simulink model "addSensorNoise"  (R2013a)
settings: Solver=ode45  StartTime=0.0  StopTime=10.0  RelTol=1e-3
values from neighbouring files (symbols this model uses):
  sampleTime = 0.01    [runPositionFilter.m]    (also in runtracklsq.m = mydata.sampleTime; workspace.mat)
libraries: simulink x9
settings Model: Creator=User  LastModifiedBy=User

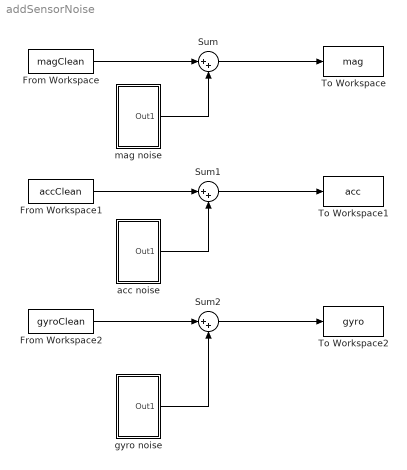
== system addSensorNoise ==
  From Workspace : FromWorkspace  VariableName=magClean  SampleTime=sampleTime
  From Workspace1 : FromWorkspace  VariableName=accClean  SampleTime=sampleTime
  From Workspace2 : FromWorkspace  VariableName=gyroClean  SampleTime=sampleTime
  Sum : Sum  Inputs=|++
  Sum1 : Sum  Inputs=|++
  Sum2 : Sum  Inputs=|++
  To Workspace : ToWorkspace  VariableName=mag  SampleTime=sampleTime  SaveFormat=Structure With Time
  To Workspace1 : ToWorkspace  VariableName=acc  SampleTime=sampleTime  SaveFormat=Structure With Time
  To Workspace2 : ToWorkspace  VariableName=gyro  SampleTime=sampleTime  SaveFormat=Structure With Time
  acc noise : Subsystem
  gyro noise : Subsystem
  "mag noise " : Subsystem
  wires:
  From Workspace/1 -> Sum/1
  Sum/1 -> To Workspace/1
  From Workspace1/1 -> Sum1/1
  Sum1/1 -> To Workspace1/1
  From Workspace2/1 -> Sum2/1
  Sum2/1 -> To Workspace2/1
  "mag noise "/1(Out1) -> Sum/2
  acc noise/1(Out1) -> Sum1/2
  gyro noise/1(Out1) -> Sum2/2

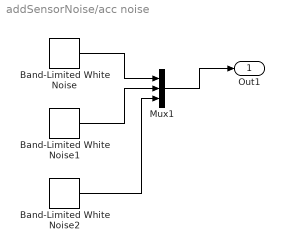
== system addSensorNoise/acc noise ==
  Band-Limited White Noise : simulink/Sources/Band-Limited White Noise  Cov=[0.001]*sampleTime*1  Ts=sampleTime  seed=[23341]
  Band-Limited White Noise1 : simulink/Sources/Band-Limited White Noise  Cov=[0.001]*sampleTime*1  Ts=sampleTime  seed=[23341]
  Band-Limited White Noise2 : simulink/Sources/Band-Limited White Noise  Cov=[0.001]*sampleTime*1  Ts=sampleTime  seed=[23341]
  Mux1 : Mux  Inputs=3
  Out1 : Outport
  wires:
  Mux1/1 -> Out1/1
  Band-Limited White Noise1/1 -> Mux1/2
  Band-Limited White Noise2/1 -> Mux1/3
  Band-Limited White Noise/1 -> Mux1/1

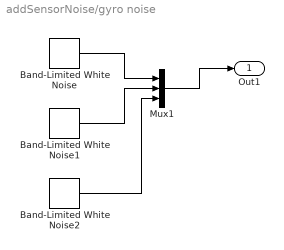
== system addSensorNoise/gyro noise ==
  Band-Limited White Noise : simulink/Sources/Band-Limited White Noise  Cov=[0.001]*sampleTime*1  Ts=sampleTime  seed=[23341]
  Band-Limited White Noise1 : simulink/Sources/Band-Limited White Noise  Cov=[0.001]*sampleTime*1  Ts=sampleTime  seed=[23341]
  Band-Limited White Noise2 : simulink/Sources/Band-Limited White Noise  Cov=[0.001]*sampleTime*1  Ts=sampleTime  seed=[23341]
  Mux1 : Mux  Inputs=3
  Out1 : Outport
  wires:
  Mux1/1 -> Out1/1
  Band-Limited White Noise1/1 -> Mux1/2
  Band-Limited White Noise2/1 -> Mux1/3
  Band-Limited White Noise/1 -> Mux1/1

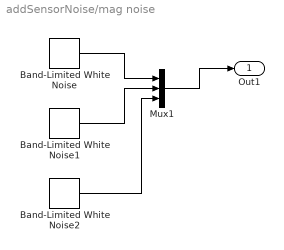
== system addSensorNoise/mag noise  ==
  Band-Limited White Noise : simulink/Sources/Band-Limited White Noise  Cov=[0.001]*sampleTime*1  Ts=sampleTime  seed=[23341]
  Band-Limited White Noise1 : simulink/Sources/Band-Limited White Noise  Cov=[0.001]*sampleTime*1  Ts=sampleTime  seed=[23341]
  Band-Limited White Noise2 : simulink/Sources/Band-Limited White Noise  Cov=[0.001]*sampleTime*1  Ts=sampleTime  seed=[23341]
  Mux1 : Mux  Inputs=3
  Out1 : Outport
  wires:
  Mux1/1 -> Out1/1
  Band-Limited White Noise1/1 -> Mux1/2
  Band-Limited White Noise2/1 -> Mux1/3
  Band-Limited White Noise/1 -> Mux1/1
